simulink model "PID_LQR_GPC"  (R2022b)
settings: Solver=ode5  StartTime=0.0  StopTime=5  FixedStep=0.01  RelTol=1e-3
values from neighbouring files (symbols this model uses):
  K = [0.06  0.0 0.0125]    [servo_start.m]
  Ks = 195    [Servo_calc_lq.m]    (also in Servo_calc_lq_d.m; servo_start.m)
  T0 = 0.01    [Servo_calc_lq.m]    (also in Servo_calc_lq_d.m; servo_start.m)
  Ts = 0.86    [Servo_calc_lq.m]    (also in Servo_calc_lq_d.m; servo_start.m)
undefined symbols (not defined in the file or in its folder): DiscIntNeverNeededParam
settings Model: Creator=artur  LastModifiedBy=artur

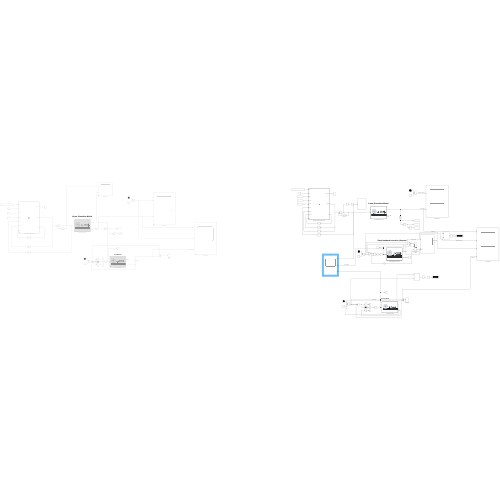
[thumbnail: Simulink's stored preview of the top-level diagram]
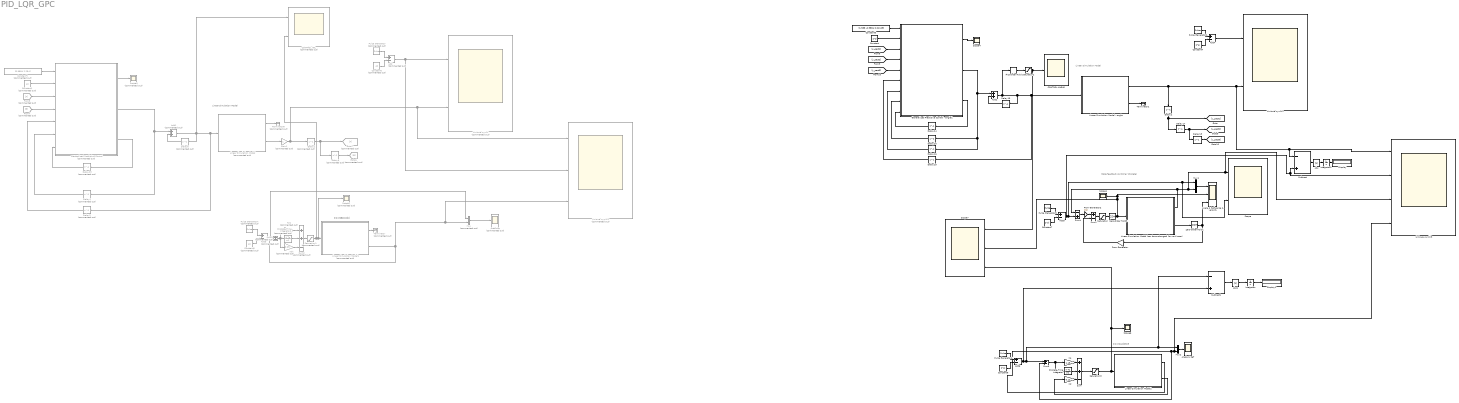
== system PID_LQR_GPC ==
  note: Linear Simulation Model
  note: PID PRĘDKOŚĆ
  note: Linear Simulation Model
  note: State feedback controller (discrete)
  note: PID POŁOŻENIE
  Abs : Abs  SaturateOnIntegerOverflow=off
  Abs1 : Abs  SaturateOnIntegerOverflow=off
  Add : Sum  Commented=on  Inputs=+-
  Add1 : Sum  Commented=on
  Add2 : Sum
  Add3 : Sum  Commented=on  Inputs=+-
  Add4 : Sum  Inputs=+-
  Add5 : Sum  Inputs=+-
  Add6 : Sum  Inputs=+-
  Angle & Ref : Scope
  Angle & Reference & velocity : Scope  NumInputPorts=3
  CONTROL ANGLE : Scope
  CONTROL VEL : Scope  Commented=on  NumInputPorts=2
  Constant{,4,7..8} (4 alike) : Constant  Value=2*pi
  Constant1 : Constant  Commented=on  Value=40
  Constant2 : Constant  Commented=on  Value=40
  Constant3 : Constant  Commented=on  Value=40
  Constant5 : Constant  Commented=on  Value=[0.9884 2.254]
  Constant6 : Constant  Value=[1.988 -0.9884 0.01129]
  Delay{1,3..6} (5 alike) : Delay  Commented=on  DelayLength=1  InitialCondition=0
  Delay{2,15..19} (6 alike) : Delay  DelayLength=1  InitialCondition=0
  Delay20 : Delay  InitialCondition=0
  Delay23 : Delay  Commented=on  DelayLength=1  InitialCondition=1
  Delay24 : Delay  DelayLength=1  InitialCondition=1
  Discrete-Time Integrator : DiscreteIntegrator  gainval=0.02  SampleTime=-1  ICPrevOutput=DiscIntNeverNeededParam  ICPrevScaledInput=DiscIntNeverNeededParam
  Discrete-Time Integrator1 : DiscreteIntegrator  Commented=on  gainval=0.05  SampleTime=-1  ICPrevOutput=DiscIntNeverNeededParam  ICPrevScaledInput=DiscIntNeverNeededParam
  Display : Display
  Display1 : Display
  First Order Hold : FirstOrderHold  ErrorTolerance=inf
  From Generator : Gain  Gain=K(2)  SaturateOnIntegerOverflow=on  OutDataTypeStr=Inherit: Same as input  ParamDataTypeStr=Inherit: Same as input
  From Generator2 : Gain  Gain=K(1)  SaturateOnIntegerOverflow=on  OutDataTypeStr=Inherit: Same as input  ParamDataTypeStr=Inherit: Same as input
  From3 : From  Commented=on
  From7 : From  Commented=on  GotoTag=B
  Gain1 : Gain  Commented=on
  Generalized Predictive Control : MATLAB Function  Commented=on  TreatAsAtomicUnit=on
  Generalized Predictive Control - angle1 : MATLAB Function  TreatAsAtomicUnit=on
  Goto6 : Goto  Commented=on  GotoTag=B
  Goto7 : Goto  Commented=on
  Integrator : Integrator
  Integrator1 : Integrator
  Kd : Gain  Gain=0.12  SaturateOnIntegerOverflow=on  OutDataTypeStr=Inherit: Same as input  ParamDataTypeStr=Inherit: Same as input
  Kd1 : Gain  Commented=on  Gain=0.05  SaturateOnIntegerOverflow=on  OutDataTypeStr=Inherit: Same as input  ParamDataTypeStr=Inherit: Same as input
  Kp : Gain  Gain=1.15  SaturateOnIntegerOverflow=on  OutDataTypeStr=Inherit: Same as input  ParamDataTypeStr=Inherit: Same as input
  Kp1 : Gain  Commented=on  Gain=1.35  SaturateOnIntegerOverflow=on  OutDataTypeStr=Inherit: Same as input  ParamDataTypeStr=Inherit: Same as input
  Linear Simulation Model : Subsystem  Commented=on  mask{x0=[0 0]}
      mask prompts: x0 "Initial conditions [angle vel]"
      mask Display: image(imread('Servo_m.JPG'))
  Linear Simulation Model (can be exchanged  for nonlinear) : Subsystem  mask{x0=[0 0]}
      mask prompts: x0 "Initial conditions [angle vel]"
      mask Display: image(imread('Servo_m.JPG'))
  Linear Simulation Model - angle : Subsystem  mask{x0=[0 0]}
      mask prompts: x0 "Initial conditions [angle vel]"
      mask Display: image(imread('Servo_m.JPG'))
  Linear Simulation Model1 : Subsystem  Commented=on  mask{x0=[0*25*pi/2 0]}
      mask prompts: x0 "Initial conditions [angle vel]"
      mask Display: image(imread('Servo_m.JPG'))
  Linear Simulation Model2 : Subsystem  mask{x0=[0*25*pi/2 0]}
      mask prompts: x0 "Initial conditions [angle vel]"
      mask Display: image(imread('Servo_m.JPG'))
  Liniowe wyniki : Scope  Commented=on  NumInputPorts=2
  Liniowe wyniki1 : Scope  NumInputPorts=2
  Liniowe wyniki2 : Scope  Commented=on  NumInputPorts=3
  Liniowe wyniki3 : Scope  NumInputPorts=4
  Mux : Mux  Commented=on  Inputs=2
  Mux1 : Mux  Inputs=2
  Mux2 : Mux  Inputs=2
  Pulse Generator : DiscretePulseGenerator  Commented=on  PulseType=Time based  Amplitude=80  Period=4  PulseWidth=50
  Pulse Generator1 : DiscretePulseGenerator  Commented=on  PulseType=Time based  Amplitude=80  Period=4  PulseWidth=50
  Pulse Generator2 : DiscretePulseGenerator  PulseType=Time based  Amplitude=4*pi  Period=4  PulseWidth=50
  Pulse Generator3 : DiscretePulseGenerator  PulseType=Time based  Amplitude=4*pi  Period=4  PulseWidth=50
  Pulse Generator4 : DiscretePulseGenerator  PulseType=Time based  Amplitude=4*pi  Period=4  PulseWidth=50
  Saturation : Saturate  UpperLimit=1  LowerLimit=-1
  Saturation1 : Saturate  Commented=on  UpperLimit=1  LowerLimit=-1
  Saturation2 : Saturate  UpperLimit=1  LowerLimit=-1
  Saturation3 : Saturate  UpperLimit=1  LowerLimit=-1
  Scope : Scope  NumInputPorts=2
  Scope1 : Scope
  Scope2 : Scope  Commented=on
  Scope3 : Scope  Commented=on
  Scope4 : Scope
  Scope6 : Scope
  Scope7 : Scope  NumInputPorts=3
  Subtract : Sum  Inputs=-+
  Subtract1 : Sum  Inputs=-+
  Sum : Sum  Inputs=++-  InputSameDT=on  SaturateOnIntegerOverflow=on  OutDataTypeStr=Inherit: Same as first input
  Sum1 : Sum  Inputs=+-  InputSameDT=on  SaturateOnIntegerOverflow=on  OutDataTypeStr=Inherit: Same as first input
  Sum2 : Sum  Commented=on  Inputs=++-  InputSameDT=on  SaturateOnIntegerOverflow=on  OutDataTypeStr=Inherit: Same as first input
  Sum3 : Sum  Commented=on  Inputs=+-  InputSameDT=on  SaturateOnIntegerOverflow=on  OutDataTypeStr=Inherit: Same as first input
  Sum4 : Sum  Inputs=-+  InputSameDT=on  SaturateOnIntegerOverflow=on  OutDataTypeStr=Inherit: Same as first input
  Sum5 : Sum  Inputs=+-  InputSameDT=on  SaturateOnIntegerOverflow=on  OutDataTypeStr=Inherit: Same as first input
  Terminator : Terminator  Commented=on
  Terminator1 : Terminator
  Terminator8 : Terminator  Commented=on
  Zero-Order Hold1 : ZeroOrderHold  SampleTime=T0
  Zero-Order Hold3 : ZeroOrderHold  SampleTime=T0
  predkosc : Scope  Commented=on
  wires:
  Delay23/1 -> Generalized Predictive Control/7(cntp)
  From3/1 -> Generalized Predictive Control/3(y_past1)
  Delay3/1 -> Generalized Predictive Control/5(u_past)
  Add/1 -> Liniowe wyniki2/2, Liniowe wyniki/1  "Trajektoria referencyjna"
  From7/1 -> Generalized Predictive Control/4(y_past2)
  Generalized Predictive Control/2(du_control) -> Delay4/1, Add1/1  "du"
  Delay4/1 -> Generalized Predictive Control/6(du_past)
  Linear Simulation Model/1(Angle) -> Terminator8/1  "Angle"
  Delay6/1 -> Add1/2
  Constant2/1 -> Add/2
  Generalized Predictive Control/3(cnt) -> Delay23/1
  Mux/1 -> predkosc/1
  Pulse Generator/1 -> Add/1
  Gain1/1 -> Delay1/1, Liniowe wyniki2/1, Liniowe wyniki/2  "Regulator GPC"
  Linear Simulation Model/2(Velocity) -> Gain1/1  "Velocity"
  Constant1/1 -> Generalized Predictive Control/2(ref)
  Add1/1 -> CONTROL VEL/1, Delay3/1, Linear Simulation Model/1(Control), Delay6/1
  Delay5/1 -> Goto6/1
  Constant5/1 -> Generalized Predictive Control/1(theta)
  Generalized Predictive Control/1(du_predicted) -> Scope3/1
  Discrete-Time Integrator1/1 -> Sum2/2
  Sum3/1 -> Discrete-Time Integrator1/1, Kp1/1, Kd1/1  "e alfa"
  Kp1/1 -> Sum2/1
  Pulse Generator1/1 -> Add3/1
  Add3/1 -> Mux/1, Sum3/1
  Sum2/1 -> Saturation1/1
  Linear Simulation Model1/1(Angle) -> Terminator/1  "Angle"
  Kd1/1 -> Sum2/3
  Linear Simulation Model1/2(Velocity) -> Liniowe wyniki2/3, Mux/2, Sum3/2  "Regulator PID"
  Constant3/1 -> Add3/2
  Saturation1/1 -> CONTROL VEL/2, Scope2/1, Linear Simulation Model1/1(Control)
  Constant6/1 -> Generalized Predictive Control - angle1/1(theta)  "ref"
  Generalized Predictive Control - angle1/2(du_control) -> Delay16/1, Delay20/1, Add2/1  "du"
  Delay19/1 -> Generalized Predictive Control - angle1/6(u_past)
  Generalized Predictive Control - angle1/1(du_predicted) -> Scope4/1
  Linear Simulation Model - angle/2(Velocity) -> Terminator1/1  "Velocity"
  Generalized Predictive Control - angle1/3(cnt) -> Delay24/1
  Add2/1 -> Delay15/1, Delay19/1, Linear Simulation Model - angle/1(Control), First Order Hold/1  "S"
  Delay16/1 -> Generalized Predictive Control - angle1/7(du_past1)
  Linear Simulation Model - angle/1(Angle) -> Delay2/1, Liniowe wyniki3/1, Subtract/1, Liniowe wyniki1/2  "Regulator GPC"
  First Order Hold/1 -> Saturation2/1
  [y_past1] -> Generalized Predictive Control - angle1/3(y_past1)
  Delay2/1 -> Delay17/1, [y_past1]
  [y_past2] -> Generalized Predictive Control - angle1/4(y_past2)
  Delay18/1 -> [y_past3]
  Constant4/1 -> Add4/2
  Delay17/1 -> Delay18/1, [y_past2]
  Delay20/1 -> Generalized Predictive Control - angle1/8(du_past2)
  Add4/1 -> Liniowe wyniki1/1  "Trajektoria referencyjna"
  Pulse Generator2/1 -> Add4/1
  Delay24/1 -> Generalized Predictive Control - angle1/9(cntp)
  Delay15/1 -> Add2/2
  Constant/1 -> Generalized Predictive Control - angle1/2(ref)
  [y_past3] -> Generalized Predictive Control - angle1/5(y_past3)
  From Generator/1 -> Sum1/2
  Add5/1 -> Liniowe wyniki3/2, Subtract/2, Sum4/2, Scope/2, Mux1/1  "Trajektoria referencyjna"
  Sum4/1 -> From Generator2/1
  Linear Simulation Model (can be exchanged  for nonlinear)/1(Angle) -> Liniowe wyniki3/3, Scope/1, Mux1/2, Sum4/1  "Regulator LQR"
  Mux1/1 -> Angle & Reference & velocity/1  "Angle & ref"
  From Generator2/1 -> Sum1/1
  Zero-Order Hold3/1 -> Scope7/2, Scope1/1, Angle & Reference & velocity/2, Linear Simulation Model (can be exchanged  for nonlinear)/1(Control)  "Regulator LQR"
  Zero-Order Hold1/1 -> Angle & Reference & velocity/3, From Generator/1
  Pulse Generator3/1 -> Add5/1
  Sum1/1 -> Saturation/1
  Saturation/1 -> Zero-Order Hold3/1
  Linear Simulation Model (can be exchanged  for nonlinear)/2(Velocity) -> Zero-Order Hold1/1  "velocity (tacho)"
  Constant7/1 -> Add5/2
  Saturation2/1 -> CONTROL ANGLE/1, Scope7/1  "Regulator MPC"
  Delay1/1 -> Delay5/1, Goto7/1
  Constant8/1 -> Add6/2
  Integrator/1 -> Display1/1
  Subtract1/1 -> Abs1/1
  Saturation3/1 -> Scope7/3, Scope6/1, Linear Simulation Model2/1(Control)  "Regulator PID"
  Discrete-Time Integrator/1 -> Sum/2
  Pulse Generator4/1 -> Add6/1
  Kd/1 -> Sum/3
  Sum/1 -> Saturation3/1
  Linear Simulation Model2/2(Velocity) -> Kd/1  "velocity"
  Add6/1 -> Subtract1/2, Sum5/1, Subtract1/1, Mux2/1  "Trajektoria referencyjna"
  Mux2/1 -> Angle & Ref/1
  Linear Simulation Model2/1(Angle) -> Sum5/2, Liniowe wyniki3/4, Mux2/2  "Regulator PID"
  Sum5/1 -> Discrete-Time Integrator/1, Kp/1  "e alfa"
  Abs1/1 -> Integrator/1
  Kp/1 -> Sum/1
  Integrator1/1 -> Display/1
  Abs/1 -> Integrator1/1
  Subtract/1 -> Abs/1

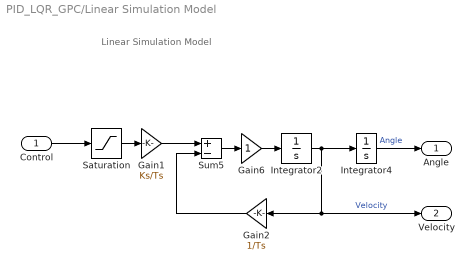
== system PID_LQR_GPC/Linear Simulation Model ==
  note: Linear Simulation Model
  Control : Inport
  Gain1 : Gain  Gain=Ks/Ts  SaturateOnIntegerOverflow=on  OutDataTypeStr=Inherit: Same as input  ParamDataTypeStr=Inherit: Same as input
  Gain2 : Gain  Gain=1/Ts  SaturateOnIntegerOverflow=on  OutDataTypeStr=Inherit: Same as input  ParamDataTypeStr=Inherit: Same as input
  Gain6 : Gain  SaturateOnIntegerOverflow=on  OutDataTypeStr=Inherit: Same as input  ParamDataTypeStr=Inherit: Same as input
  Integrator2 : Integrator  InitialCondition=x0(2)
  Integrator4 : Integrator  InitialCondition=x0(1)
  Saturation : Saturate  UpperLimit=1  LowerLimit=-1
  Sum5 : Sum  Inputs=+-  InputSameDT=on  SaturateOnIntegerOverflow=on  OutDataTypeStr=Inherit: Same as first input
  Angle : Outport  InitialOutput=0  VectorParamsAs1DForOutWhenUnconnected=off
  Velocity : Outport  Port=2  InitialOutput=0  VectorParamsAs1DForOutWhenUnconnected=off
  wires:
  Sum5/1 -> Gain6/1
  Gain2/1 -> Sum5/2
  Integrator2/1 -> Integrator4/1, Velocity/1, Gain2/1  "Velocity"
  Integrator4/1 -> Angle/1  "Angle"
  Gain6/1 -> Integrator2/1
  Control/1 -> Saturation/1
  Saturation/1 -> Gain1/1
  Gain1/1 -> Sum5/1

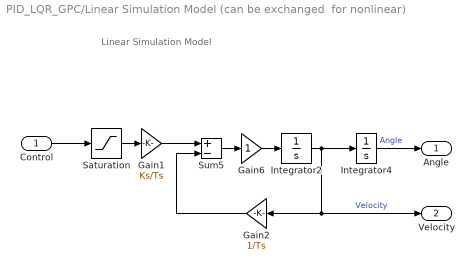
== system PID_LQR_GPC/Linear Simulation Model (can be exchanged  for nonlinear) ==
  note: Linear Simulation Model
  Control : Inport
  Gain1 : Gain  Gain=Ks/Ts  SaturateOnIntegerOverflow=on  OutDataTypeStr=Inherit: Same as input  ParamDataTypeStr=Inherit: Same as input
  Gain2 : Gain  Gain=1/Ts  SaturateOnIntegerOverflow=on  OutDataTypeStr=Inherit: Same as input  ParamDataTypeStr=Inherit: Same as input
  Gain6 : Gain  SaturateOnIntegerOverflow=on  OutDataTypeStr=Inherit: Same as input  ParamDataTypeStr=Inherit: Same as input
  Integrator2 : Integrator  InitialCondition=x0(2)
  Integrator4 : Integrator  InitialCondition=x0(1)
  Saturation : Saturate  UpperLimit=1  LowerLimit=-1
  Sum5 : Sum  Inputs=+-  InputSameDT=on  SaturateOnIntegerOverflow=on  OutDataTypeStr=Inherit: Same as first input
  Angle : Outport  InitialOutput=0  VectorParamsAs1DForOutWhenUnconnected=off
  Velocity : Outport  Port=2  InitialOutput=0  VectorParamsAs1DForOutWhenUnconnected=off
  wires:
  Gain1/1 -> Sum5/1
  Saturation/1 -> Gain1/1
  Control/1 -> Saturation/1
  Gain6/1 -> Integrator2/1
  Integrator4/1 -> Angle/1  "Angle"
  Integrator2/1 -> Gain2/1, Velocity/1, Integrator4/1  "Velocity"
  Gain2/1 -> Sum5/2
  Sum5/1 -> Gain6/1

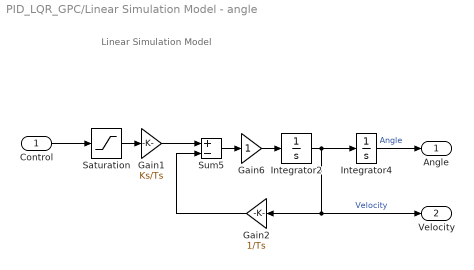
== system PID_LQR_GPC/Linear Simulation Model - angle ==
  note: Linear Simulation Model
  Control : Inport
  Gain1 : Gain  Gain=Ks/Ts  SaturateOnIntegerOverflow=on  OutDataTypeStr=Inherit: Same as input  ParamDataTypeStr=Inherit: Same as input
  Gain2 : Gain  Gain=1/Ts  SaturateOnIntegerOverflow=on  OutDataTypeStr=Inherit: Same as input  ParamDataTypeStr=Inherit: Same as input
  Gain6 : Gain  SaturateOnIntegerOverflow=on  OutDataTypeStr=Inherit: Same as input  ParamDataTypeStr=Inherit: Same as input
  Integrator2 : Integrator  InitialCondition=x0(2)
  Integrator4 : Integrator  InitialCondition=x0(1)
  Saturation : Saturate  UpperLimit=1  LowerLimit=-1
  Sum5 : Sum  Inputs=+-  InputSameDT=on  SaturateOnIntegerOverflow=on  OutDataTypeStr=Inherit: Same as first input
  Angle : Outport  InitialOutput=0  VectorParamsAs1DForOutWhenUnconnected=off
  Velocity : Outport  Port=2  InitialOutput=0  VectorParamsAs1DForOutWhenUnconnected=off
  wires:
  Sum5/1 -> Gain6/1
  Gain2/1 -> Sum5/2
  Integrator2/1 -> Integrator4/1, Velocity/1, Gain2/1  "Velocity"
  Integrator4/1 -> Angle/1  "Angle"
  Gain6/1 -> Integrator2/1
  Control/1 -> Saturation/1
  Saturation/1 -> Gain1/1
  Gain1/1 -> Sum5/1

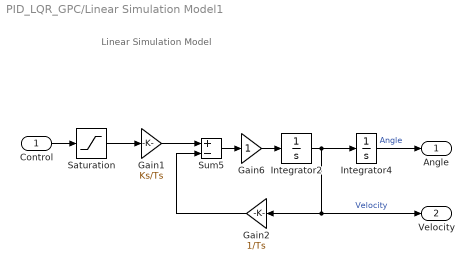
== system PID_LQR_GPC/Linear Simulation Model1 ==
  note: Linear Simulation Model
  Control : Inport
  Gain1 : Gain  Gain=Ks/Ts  SaturateOnIntegerOverflow=on  OutDataTypeStr=Inherit: Same as input  ParamDataTypeStr=Inherit: Same as input
  Gain2 : Gain  Gain=1/Ts  SaturateOnIntegerOverflow=on  OutDataTypeStr=Inherit: Same as input  ParamDataTypeStr=Inherit: Same as input
  Gain6 : Gain  SaturateOnIntegerOverflow=on  OutDataTypeStr=Inherit: Same as input  ParamDataTypeStr=Inherit: Same as input
  Integrator2 : Integrator  InitialCondition=x0(2)
  Integrator4 : Integrator  InitialCondition=x0(1)
  Saturation : Saturate  UpperLimit=1  LowerLimit=-1
  Sum5 : Sum  Inputs=+-  InputSameDT=on  SaturateOnIntegerOverflow=on  OutDataTypeStr=Inherit: Same as first input
  Angle : Outport  InitialOutput=0  VectorParamsAs1DForOutWhenUnconnected=off
  Velocity : Outport  Port=2  InitialOutput=0  VectorParamsAs1DForOutWhenUnconnected=off
  wires:
  Sum5/1 -> Gain6/1
  Gain2/1 -> Sum5/2
  Integrator2/1 -> Integrator4/1, Velocity/1, Gain2/1  "Velocity"
  Integrator4/1 -> Angle/1  "Angle"
  Gain6/1 -> Integrator2/1
  Control/1 -> Saturation/1
  Gain1/1 -> Sum5/1
  Saturation/1 -> Gain1/1

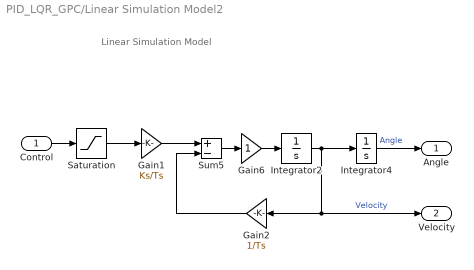
== system PID_LQR_GPC/Linear Simulation Model2 ==
  note: Linear Simulation Model
  Control : Inport
  Gain1 : Gain  Gain=Ks/Ts  SaturateOnIntegerOverflow=on  OutDataTypeStr=Inherit: Same as input  ParamDataTypeStr=Inherit: Same as input
  Gain2 : Gain  Gain=1/Ts  SaturateOnIntegerOverflow=on  OutDataTypeStr=Inherit: Same as input  ParamDataTypeStr=Inherit: Same as input
  Gain6 : Gain  SaturateOnIntegerOverflow=on  OutDataTypeStr=Inherit: Same as input  ParamDataTypeStr=Inherit: Same as input
  Integrator2 : Integrator  InitialCondition=x0(2)
  Integrator4 : Integrator  InitialCondition=x0(1)
  Saturation : Saturate  UpperLimit=1  LowerLimit=-1
  Sum5 : Sum  Inputs=+-  InputSameDT=on  SaturateOnIntegerOverflow=on  OutDataTypeStr=Inherit: Same as first input
  Angle : Outport  InitialOutput=0  VectorParamsAs1DForOutWhenUnconnected=off
  Velocity : Outport  Port=2  InitialOutput=0  VectorParamsAs1DForOutWhenUnconnected=off
  wires:
  Sum5/1 -> Gain6/1
  Gain2/1 -> Sum5/2
  Integrator2/1 -> Integrator4/1, Velocity/1, Gain2/1  "Velocity"
  Integrator4/1 -> Angle/1  "Angle"
  Gain6/1 -> Integrator2/1
  Control/1 -> Saturation/1
  Gain1/1 -> Sum5/1
  Saturation/1 -> Gain1/1

== matlab function PID_LQR_GPC/Generalized Predictive Control ==
  data: du_predicted output; theta input; ref input; y_past1 input; y_past2 input; u_past input; du_past input; du_control output; cntp input; cnt output
function [du_predicted, du_control,cnt] = fcn(theta,ref,y_past1,y_past2,u_past,du_past,cntp)

cnt = cntp;

%Współczynniki modelu z algorytmu RLS
a1 = -theta(1);
b1 = theta(2);

%Przeszłe wyjścia
y_past = [y_past1;y_past2];
    
%Parametry
ny = 120; %HORYZONT PREDYKCJI
nu = 48; %HORYZONT STEROWANIA
lambda = 0.5;
    
%Czy wykorzystać T-filtr?
filtrowanie = false;
    
%Ustawienie ograniczeń dla optymalizatora 
%true - ograniczenia na y, false - bez ograniczeń na y
ograniczenie_wyjscia = true;

du_max = 1;
du_min = -1;
u_max = 1;
u_min = -1;
y_max = 42;
y_min = -42;

%Trajektoria referencyjna, stała
Ts = 0.01; %PRÓBKOWANIE SYMULACJI
sim_time = 4; %CZAS SYMULACJI

traj_ub = ref*ones(1/Ts*sim_time/2,1);

traj_lb = -ref*ones(1/Ts*sim_time/2,1);

trajektoria = [traj_ub;traj_lb;traj_ub;-ref*ones(ny,1)];

ref = trajektoria(cnt:ny+cnt-1, 1);

cnt = cntp + 1;

%%%



    %Wyznaczenie wielomianów a i b
    a = [1 a1];
    b = [0 b1];
    A = conv(a,[1 -1]);
    
    %Wyznaczenie macierzy predykcji
    [Ca,Ha] = predmat(A,ny);
    [Cb,Hb] = predmat(b,ny);
    
    Cai = inv(Ca);
    
    H = Cai*Cb;
    P = Cai*Hb;
    Q = Cai*(-Ha);

%%%%%%%%%%%%%%%%%%%%%%%%%%%%%%%%%%%%%%%%%%%%%%%%%%%%%%%%%%%%%%%%%%%%%%%%%%%

if filtrowanie == true
    Tfilt = [1 -0.2];
    
    [Ct,Ht] = predmat(Tfilt,ny);
    Pt = Ct * P - H * Ht;
    Qt = Ct * Q + Ht;
    
    P = Pt;
    Q = Qt;
end

%%%%%%%%%%%%%%%%%%%%%%%%%%%%%%%%%%%%%%%%%%%%%%%%%%%%%%%%%%%%%%%%%%%%%%%%%%%

    Hu = H(:,1:nu); %horyzont sterowania

%Prawo sterowania dla algorytmu z ograniczeniami
    S = Hu'*Hu + eye(nu)*lambda;
    S = (S + S')/2;
    f = Hu'*Q * y_past + Hu'*P * du_past - Hu' * ref;

    if ograniczenie_wyjscia == true
        %OGRANICZENIA Z Y
        [C,dd,du,ddu,dy] = mpc_ograniczenia(du_max, du_min,u_max,u_min,y_max,y_min,nu,Hu,P,Q,1,2);
        dt = dd + du * u_past + ddu * du_past + dy*y_past;
    else
        %OGRANICZENIA BEZ Y
        [C, dd,du] = mpc_ograniczenia_bez_y(du_max,du_min,u_max,u_min,nu);
        dt = dd + du * u_past;
    end


    opts = optimoptions('quadprog','Algorithm','active-set');

    x0 = 0.1*eye(nu,1);

    du_predicted = quadprog(S,f,C,dt,[],[],[],[],x0,opts);

    du_control = du_predicted(1);


%Prawo sterowania dla algorytmu bez ograniczeń
% Pr = ( inv(Hu'*Hu+lambda*eye(nu)) ) * Hu';
% Nk = Pr*Q;
% Dk = Pr*P;
% 
% du_predicted = Pr * ref - Dk * du_past - Nk*y_past;
% du_control = du_predicted(1);

== matlab function PID_LQR_GPC/Generalized Predictive Control - angle1 ==
  data: du_predicted output; theta input; ref input; y_past1 input; y_past2 input; y_past3 input; u_past input; du_past1 input; du_control output; du_past2 input; cnt output; cntp input
function [du_predicted, du_control,cnt] = fcn(theta,ref,y_past1,y_past2,y_past3,u_past,du_past1,du_past2,cntp)

cnt = cntp;

%Współczynniki modelu z algorytmu RLS
a1 = -theta(1);
a2 = -theta(2);
b1 = theta(3);

%Parametry
ny = 24; %HORYZONT PREDYKCJI
nu = 12; %HORYZONT STEROWANIA
lambda = 0.5;

%Przeszłe wyjścia
y_past = [y_past1;y_past2;y_past3];
du_past = [du_past1;du_past2];

%Trajektoria referencyjna, stała

%Trajektoria referencyjna, stała
Ts = 0.01; %PRÓBKOWANIE SYMULACJI
sim_time = 4; %CZAS SYMULACJI

traj_ub = ref*ones(1/Ts*sim_time/2,1);

traj_lb = -ref*ones(1/Ts*sim_time/2,1);

%%% trajektoria referencyjna
trajektoria = [traj_ub;traj_lb;traj_ub;-ref*ones(ny,1)];

ref = trajektoria(cnt:ny+cnt-1, 1);

cnt = cntp + 1;

%%%

%Czy wykorzystać T-filtr?
filtrowanie = false;

%Ograniczenia
%true - ograniczenia na y, false - bez ograniczeń na y
ograniczenie_wyjscia = true;

du_max = 1;
du_min = -1;
u_max = 1;
u_min = -1;
y_max = 6.6;
y_min = -6.6;

%Wyznaczenie wielomianów a i b
a = [1 a1 a2];
b = [0 0 b1];
A = conv(a,[1 -1]);

%Wyznaczenie macierzy predykcji
[Ca,Ha] = predmat(A,ny);
[Cb,Hb] = predmat(b,ny);

Cai = inv(Ca);

H = Cai*Cb;
P = Cai*Hb;
Q = Cai*(-Ha);

%%%%%%%%%%%%%%%%%%%%%%%%%%%%%%%%%%%%%%%%%%%%%%%%%%%%%%%%%%%%%%%%%%%%%%%%%%%

if filtrowanie == true
    Tfilt = [1 -0.05];
    
    [Ct,Ht] = predmat(Tfilt,ny);
    Pfilt = Ct * P - H * Ht;
    Qfilt = Ct * Q + Ht;
    
    P = Pfilt;
    Q = Qfilt;
end

%%%%%%%%%%%%%%%%%%%%%%%%%%%%%%%%%%%%%%%%%%%%%%%%%%%%%%%%%%%%%%%%%%%%%%%%%%%

Hu = H(:,1:nu); %horyzont sterowania

%Ustawienie ograniczeń dla optymalizatora 

%Prawo sterowania dla algorytmu z ograniczeniami
S = Hu'*Hu + eye(nu)*lambda;
S = (S + S')/2;
f = Hu'*Q * y_past + Hu'*P * du_past - Hu' * ref;

    if ograniczenie_wyjscia == true
        %OGRANICZENIA Z Y
        [C,dd,du,ddu,dy] = mpc_ograniczenia(du_max, du_min,u_max,u_min,y_max,y_min,nu,Hu,P,Q,2,3);
        dt = dd + du * u_past + ddu * du_past + dy*y_past;
    else
        %OGRANICZENIA BEZ Y
        [C, dd,du] = mpc_ograniczenia_bez_y(du_max,du_min,u_max,u_min,nu);
        dt = dd + du * u_past;
    end


opts = optimoptions('quadprog','Algorithm','active-set');

x0 = 0*eye(nu,1);

du_predicted = quadprog(S,f,C,dt,[],[],[],[],x0,opts);

du_control = du_predicted(1);

%Prawo sterowania dla algorytmu bez ograniczeń
% Pr = ( inv(Hu'*Hu+lambda*eye(nu)) ) * Hu';
% Nk = Pr*Q;
% Dk = Pr*P;
% 
% du_predicted = Pr * ref - Dk * du_past - Nk*y_past;
% du_control = du_predicted(1);
